simulink model "turbin"  (R2013a)
settings: Solver=ode45  StartTime=0.0  StopTime=10.0  RelTol=1e-3
values from neighbouring files (symbols this model uses):
  cp_exh = gamma_exh*cv_exh    (= 980)    [Init_Project1.m]
  T_amb = 293    [Init_Project1.m]
  T_em = mean(T_em)    [Init_Project1.m]    (also in Init_Project2.m = mean(T_t*(1-eta_T.*(1-Pi_T.^((gamma_exh-1)/gamma_exh)))))
  TFP_exp = turbine_parameters(2)    [Init_Project2.m]
  TFP_max = turbine_parameters(1)    [Init_Project2.m]
settings Model: Creator=rasme879  LastModifiedBy=rasme879

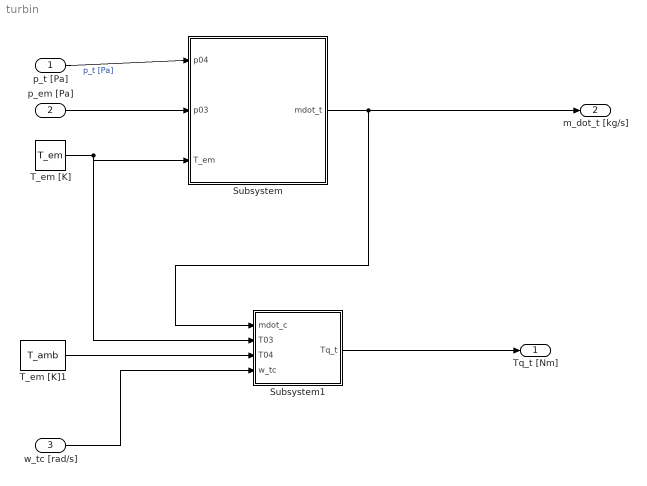
== system turbin ==
  "p_t [Pa] " : Inport
  p_em [Pa] : Inport  Port=2
  w_tc [rad/s] : Inport  Port=3
  Subsystem : Subsystem
  Subsystem1 : Subsystem
  T_em [K] : Constant  Value=T_em
  T_em [K]1 : Constant  Value=T_amb
  Tq_t [Nm] : Outport
  m_dot_t [kg/s] : Outport  Port=2
  wires:
  p_em [Pa]/1 -> Subsystem/2(p03)
  "p_t [Pa] "/1 -> Subsystem/1(p04)  "p_t [Pa]"
  T_em [K]/1 -> Subsystem1/2(T03), Subsystem/3(T_em)
  Subsystem/1(mdot_t) -> Subsystem1/1(mdot_c), m_dot_t [kg/s]/1
  w_tc [rad/s]/1 -> Subsystem1/4(w_tc)
  Subsystem1/1(Tq_t) -> Tq_t [Nm]/1
  T_em [K]1/1 -> Subsystem1/3(T04)

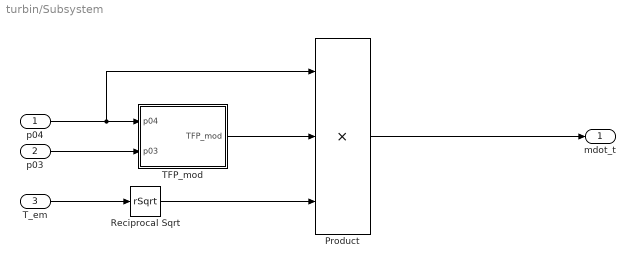
== system turbin/Subsystem ==
  p04 : Inport
  p03 : Inport  Port=2
  T_em : Inport  Port=3
  Product : Product  Inputs=3
  Reciprocal Sqrt : Sqrt  Operator=rSqrt  SaturateOnIntegerOverflow=on
  TFP_mod : Subsystem
  mdot_t : Outport
  wires:
  Reciprocal Sqrt/1 -> Product/3
  T_em/1 -> Reciprocal Sqrt/1
  TFP_mod/1(TFP_mod) -> Product/2
  p03/1 -> TFP_mod/2(p03)
  Product/1 -> mdot_t/1
  p04/1 -> Product/1, TFP_mod/1(p04)

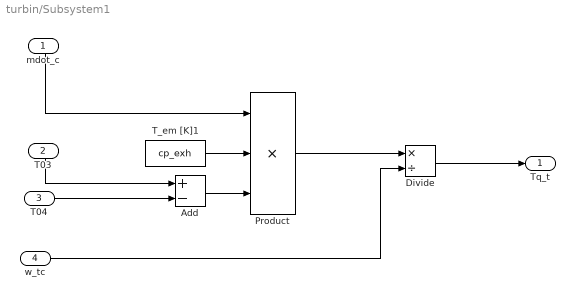
== system turbin/Subsystem1 ==
  mdot_c : Inport
  T03 : Inport  Port=2
  T04 : Inport  Port=3
  w_tc : Inport  Port=4
  Add : Sum  Inputs=+-
  Divide : Product  Inputs=*/
  Product : Product  Inputs=3
  T_em [K]1 : Constant  Value=cp_exh
  Tq_t : Outport
  wires:
  T03/1 -> Add/1
  Add/1 -> Product/3
  w_tc/1 -> Divide/2
  Divide/1 -> Tq_t/1
  Product/1 -> Divide/1
  T_em [K]1/1 -> Product/2
  mdot_c/1 -> Product/1
  T04/1 -> Add/2

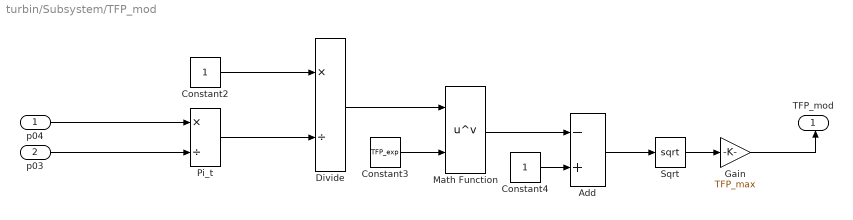
== system turbin/Subsystem/TFP_mod ==
  p04 : Inport
  p03 : Inport  Port=2
  Add : Sum  Inputs=-+
  Constant2 : Constant
  Constant3 : Constant  Value=TFP_exp
  Constant4 : Constant
  Divide : Product  Inputs=*/
  Gain : Gain  Gain=TFP_max
  Math Function : Math  Operator=pow  SaturateOnIntegerOverflow=on
  Pi_t : Product  Inputs=*/
  Sqrt : Sqrt  SaturateOnIntegerOverflow=on
  TFP_mod : Outport
  wires:
  p03/1 -> Pi_t/2
  p04/1 -> Pi_t/1
  Constant2/1 -> Divide/1
  Add/1 -> Sqrt/1
  Pi_t/1 -> Divide/2
  Divide/1 -> Math Function/1
  Constant3/1 -> Math Function/2
  Constant4/1 -> Add/2
  Gain/1 -> TFP_mod/1
  Sqrt/1 -> Gain/1
  Math Function/1 -> Add/1
